simulink model "vi_du_1"  (R2015a)
settings: Solver=ode4  SolverMode=SingleTasking  StartTime=0.0  StopTime=40  FixedStep=0.001  RelTol=1e-3
settings Model: CovMetricSettings=dwe  CovHtmlReporting=off  covSaveCumulativeToWorkspaceVar=off  CovSaveSingleToWorkspaceVar=off  CovExternalEMLEnable=on  Creator=ryell  LastModifiedBy=ryell
settings DataIOCC: LimitDataPoints=off  SaveFormat=Dataset
settings DebuggingCC: SFUnexpectedBacktrackingDiag=error  SFNoUnconditionalDefaultTransitionDiag=error
settings HardwareCC: ProdBitPerPointer=64  ProdLargestAtomicFloat=Float  ProdIntDivRoundTo=Zero  ProdEndianess=LittleEndian  ProdHWDeviceType=Specified
settings ModelReferenceCC: PropagateSignalLabelsOutOfModel=on
settings GRTTargetCC: TargetLangStandard=C99 (ISO)  GeneratePreprocessorConditionals=Use local settings

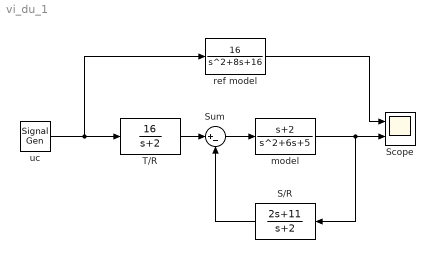
== system vi_du_1 ==
  S/R : TransferFcn  Numerator=[2 11]  Denominator=[1 2]
  Scope : Scope  NumInputPorts=2
      settings: TimeRange=auto  ShowLegends=on  MaxDataPoints=5000  SaveToWorkspace=off  SaveName=ScopeData  YMin=-1.97334~-5  YMax=1.97353~5  SampleTime=-1
  Sum : Sum  Inputs=|+-
  T/R : TransferFcn  Numerator=[16]  Denominator=[1 2]
  model : TransferFcn  Numerator=[1 2]  Denominator=[1 6 5]
  ref model : TransferFcn  Numerator=[16]  Denominator=[1 8 16]
  uc : SignalGenerator  WaveForm=square  Frequency=0.1
  wires:
  uc/1 -> ref model/1, T/R/1
  T/R/1 -> Sum/1
  Sum/1 -> model/1
  model/1 -> Scope/2, S/R/1
  S/R/1 -> Sum/2
  ref model/1 -> Scope/1
